simulink model "ES105A_StHlthSigNormn"  (R2013b)
settings: Solver=FixedStepDiscrete  SolverMode=SingleTasking  StartTime=0.0  StopTime=1  FixedStep=0.002  RelTol=1e-3
undefined symbols (not defined in the file): ARCHGLBPRM_FLOATZEROTHD_ULS_F32, CurrMeasCorrlnMaxErrCurr, CURRMOTSUMDIVBYZEROPROTNVAL_AMPR_F32, DIGTQDIVBYZEROPROTNVAL_HWNWTMTR_F32, DutyCycThermProtnDutyCycFildThd, EcuTMeasRngDiagcMax, EcuTMeasRngDiagcMin, EotLrngAuthyStrtLrn, FRICESTIMNDIVBYZEROPROTNVAL_HWNWTMTR_F32, HLTH0PERC_CNT_U08, HLTH100PERC_CNT_F32, HLTH100PERC_CNT_U08, HLTH50PERC_CNT_U08, HwTqCorrlnChATraSumSetFltThd, HwTqCorrlnChBTraSumSetFltThd, HWTQIDPTSIG_CNT_U08, MOTAG2MEAS_VALMAXERR_VOLTSQD_F32, MOTAG2MEAS_VALMINERR_VOLTSQD_F32, MOTAGCORRLN_MOTAGCORRLNERRTHD_MOTREVELEC_U0P16, MotDrvDiagcErrThd, MOTPOS2DIVBYZEROPROTNVAL2_VOLTSQD_F32, MOTPOS2DIVBYZEROPROTNVAL_VOLTSQD_F32, MOTPOSNERRDIVBYZEROPROTNVAL_MOTREV_U16, MOTPOSNERRZEROTHD_MOTREV_U0P16, NtcNr1, NtcSts1, PHAVLTGDIVBYZEROPROTNVAL_NANOSEC_F32, SigQlfr1, STHLTHSCAGFAC_CNT_F32, StHlthSigNormnAbsltMotPosDifStHlthDiagThd, StHlthSigNormnCurrMotSumStHlthDiagThd, StHlthSigNormnDigTqStHlthDiagThd, StHlthSigNormnDutyCycFltLimThd, StHlthSigNormnHiCtrlrT, StHlthSigNormnIdptSigStHlthSca, StHlthSigNormnLoCtrlrT, StHlthSigNormnMaxFricThd, StHlthSigNormnMinRackTrvlLim, StHlthSigNormnMotPosStHlthDiagThd, StHlthSigNormnMotVelCal, StHlthSigNormnPhaInfoStHlthDiagThd, StHlthSigNormnStHlthCorrlnErr, StHlthSigNormnStHlthCurrMotSum, StHlthSigNormnStHlthPhaInfo, StHlthSigNormnValMaxStHlthErr, StHlthSigNormnValMinStHlthErr, StHlthSigNormnWhlImbRejctnThd, SysGlbPrmMotPoleCnt, TSTHLTH0PERC_CNT_U08, u2, u3, u4, VLTGSTHLTH0PERC_CNT_U08
libraries: NxtrLim x39, simulink x33, NxtrAbslt x4
(part 5 of 10)

== system ES105A_StHlthSigNormn/StHlthSigNormn/UpdRawSig/Motor Position Error /AbsltMotPosBCDifStHlth Calc ==
  MotAgBCErrTerm : Inport
  Action Port : ActionPort  ActionType=default
  Constant4 : Constant  Value=StHlthSigNormnStHlthCorrlnErr
  CopyRight2 : Subsystem  Description=|  mask(Copyright Information){none=on}
      | Copyright info block.                                               
      |                                                                     
      | Place copyright information at the top of every subsystem in design.
      mask prompts: none "No parameters"
      mask help: Place copyright information at the top of every subsystem in design.
      mask Display:
      | NxtrConf = 'Nexteer Confidential';
      | 
      | sys = bdroot; %handle for the current model ("system")
      | first = get_param(sys,'Created');
      | first = first(end-3:end);  %year is last four digits
      | 
      | last = get_param(sys,'LastModifiedDate');
      | if isempty(last)
      |     last = datestr(now,'yyyy');
      | else
      |     last = last(end-3:end);
      | end
      | 
      | if strcmp(first,last)
      |     fprintf('%s -- Copyright %s Nexteer',NxtrConf,first)
      | else
      |     fprintf('%s -- %s%s- %s Nexteer',NxtrConf,char(169),first,last)
      | end
  If Action Subsystem8 : Subsystem  TreatAsAtomicUnit=on
  If Action Subsystem9 : Subsystem  TreatAsAtomicUnit=on
  If4 : If  IfExpression=u1
  LimStat_u3 : NxtrLim/LimStat_u08  LoLim=AbsltMotPosBCDifStHlth.EngMin  HiLim=AbsltMotPosBCDifStHlth.EngMax
      settings: AttributesFormatString=|
      | Low Limit: %<LoLim>
      | High Limit:%<HiLim>
  Merge2 : Merge
  Relational Operator4 : RelationalOperator  Operator=>  OutDataTypeStr=boolean
  AbsltMotPosBCDifStHlth : Outport  InitialOutput=HLTH100PERC_CNT_U08
      settings: AttributesFormatString=Initial Output: %<InitialOutput>
  wires:
  MotAgBCErrTerm/1 -> [MotAgBCErrTerm], Relational Operator4/1
  Constant4/1 -> Relational Operator4/2
  Relational Operator4/1 -> If4/1
  If4/1 -> If Action Subsystem8/Action
  If4/2 -> If Action Subsystem9/Action
  [MotAgBCErrTerm] -> If Action Subsystem8/1(MotAgBCErrTerm)
  If Action Subsystem8/1(AbsltMotPosBCDiffStHlth) -> Merge2/1
  If Action Subsystem9/1(AbsMotPosBCDiffStHlth) -> Merge2/2
  Merge2/1 -> LimStat_u3/1
  LimStat_u3/1 -> AbsltMotPosBCDifStHlth/1

== system ES105A_StHlthSigNormn/StHlthSigNormn/UpdRawSig/Motor Position Error /AbsltMotPosPhaDifStHlth ==
  NtcNr : Inport
  NtcStInfo : Inport  Port=2
  NtcSts : Inport  Port=3
  DebStep : Inport  Port=4
  SetNtcSts : Subsystem  RequirementInfo={} %GIDa_9ce26d92_e01b_4533_9a71_48efc3340490  TreatAsAtomicUnit=on
      settings: RTWSystemCode=Inline
  wires:
  NtcNr/1 -> SetNtcSts/1(NtcNr)  "NtcNr"
  NtcSts/1 -> SetNtcSts/3(NtcSts)
  DebStep/1 -> SetNtcSts/4(DebStep)
  NtcStInfo/1 -> SetNtcSts/2(NtcStInfo)

== system ES105A_StHlthSigNormn/StHlthSigNormn/UpdRawSig/Motor Position Error /CopyRight2 ==

== system ES105A_StHlthSigNormn/StHlthSigNormn/UpdRawSig/Motor Position Error /NTC Sts Calculation ==
  StHlthErr : Inport
  CopyRight2 : Subsystem  Description=|  mask(Copyright Information){none=on}
      | Copyright info block.                                               
      |                                                                     
      | Place copyright information at the top of every subsystem in design.
      mask prompts: none "No parameters"
      mask help: Place copyright information at the top of every subsystem in design.
      mask Display:
      | NxtrConf = 'Nexteer Confidential';
      | 
      | sys = bdroot; %handle for the current model ("system")
      | first = get_param(sys,'Created');
      | first = first(end-3:end);  %year is last four digits
      | 
      | last = get_param(sys,'LastModifiedDate');
      | if isempty(last)
      |     last = datestr(now,'yyyy');
      | else
      |     last = last(end-3:end);
      | end
      | 
      | if strcmp(first,last)
      |     fprintf('%s -- Copyright %s Nexteer',NxtrConf,first)
      | else
      |     fprintf('%s -- %s%s- %s Nexteer',NxtrConf,char(169),first,last)
      | end
  If : If  IfExpression=u1
  Merge : Merge
  NtcFaild : Subsystem  TreatAsAtomicUnit=on
  NtcPassd : Subsystem  TreatAsAtomicUnit=on
  NtcSts : Outport
  wires:
  StHlthErr/1 -> If/1
  If/1 -> NtcFaild/Action
  Merge/1 -> NtcSts/1
  NtcPassd/1(NtcPassd) -> Merge/2
  If/2 -> NtcPassd/Action
  NtcFaild/1(NtcFaild) -> Merge/1

== system ES105A_StHlthSigNormn/StHlthSigNormn/UpdRawSig/Phase Voltage Verification/CopyRight2 ==

== system ES105A_StHlthSigNormn/StHlthSigNormn/UpdRawSig/Phase Voltage Verification/NTC Sts Calculation ==
  StHlthErr : Inport
  CopyRight2 : Subsystem  Description=|  mask(Copyright Information){none=on}
      | Copyright info block.                                               
      |                                                                     
      | Place copyright information at the top of every subsystem in design.
      mask prompts: none "No parameters"
      mask help: Place copyright information at the top of every subsystem in design.
      mask Display:
      | NxtrConf = 'Nexteer Confidential';
      | 
      | sys = bdroot; %handle for the current model ("system")
      | first = get_param(sys,'Created');
      | first = first(end-3:end);  %year is last four digits
      | 
      | last = get_param(sys,'LastModifiedDate');
      | if isempty(last)
      |     last = datestr(now,'yyyy');
      | else
      |     last = last(end-3:end);
      | end
      | 
      | if strcmp(first,last)
      |     fprintf('%s -- Copyright %s Nexteer',NxtrConf,first)
      | else
      |     fprintf('%s -- %s%s- %s Nexteer',NxtrConf,char(169),first,last)
      | end
  If : If  IfExpression=u1
  Merge : Merge
  NtcFaild : Subsystem  TreatAsAtomicUnit=on
  NtcPassd : Subsystem  TreatAsAtomicUnit=on
  NtcSts : Outport
  wires:
  StHlthErr/1 -> If/1
  If/1 -> NtcFaild/Action
  Merge/1 -> NtcSts/1
  NtcPassd/1(NtcPassd) -> Merge/2
  If/2 -> NtcPassd/Action
  NtcFaild/1(NtcFaild) -> Merge/1

== system ES105A_StHlthSigNormn/StHlthSigNormn/UpdRawSig/Phase Voltage Verification/PhaAStHlth Calc ==
  MotDrvErrA : Inport
  Action Port : ActionPort  ActionType=case
  Constant : Constant  Value=StHlthSigNormnStHlthPhaInfo
  CopyRight2 : Subsystem  Description=|  mask(Copyright Information){none=on}
      | Copyright info block.                                               
      |                                                                     
      | Place copyright information at the top of every subsystem in design.
      mask prompts: none "No parameters"
      mask help: Place copyright information at the top of every subsystem in design.
      mask Display:
      | NxtrConf = 'Nexteer Confidential';
      | 
      | sys = bdroot; %handle for the current model ("system")
      | first = get_param(sys,'Created');
      | first = first(end-3:end);  %year is last four digits
      | 
      | last = get_param(sys,'LastModifiedDate');
      | if isempty(last)
      |     last = datestr(now,'yyyy');
      | else
      |     last = last(end-3:end);
      | end
      | 
      | if strcmp(first,last)
      |     fprintf('%s -- Copyright %s Nexteer',NxtrConf,first)
      | else
      |     fprintf('%s -- %s%s- %s Nexteer',NxtrConf,char(169),first,last)
      | end
  If : If  IfExpression=u1
  If Action Subsystem : Subsystem  TreatAsAtomicUnit=on
  If Action Subsystem1 : Subsystem  TreatAsAtomicUnit=on
  LimStat_u2 : NxtrLim/LimStat_u08  LoLim=PhaAStHlth.EngMin  HiLim=PhaAStHlth.EngMax
      settings: AttributesFormatString=|
      | Low Limit: %<LoLim>
      | High Limit:%<HiLim>
  Merge : Merge
  Relational Operator : RelationalOperator  Operator=>  OutDataTypeStr=boolean
  PhaAStHlth : Outport  InitialOutput=HLTH100PERC_CNT_U08
      settings: AttributesFormatString=Initial Output: %<InitialOutput>
  wires:
  MotDrvErrA/1 -> [MotDrvErrA], Relational Operator/1
  Constant/1 -> Relational Operator/2
  Relational Operator/1 -> If/1
  If/1 -> If Action Subsystem/Action
  If/2 -> If Action Subsystem1/Action
  [MotDrvErrA] -> If Action Subsystem/1(MotDrvErrA)
  If Action Subsystem/1(PhaseAStHlth) -> Merge/1
  If Action Subsystem1/1(PhaseAStHlth) -> Merge/2
  LimStat_u2/1 -> PhaAStHlth/1
  Merge/1 -> LimStat_u2/1

== system ES105A_StHlthSigNormn/StHlthSigNormn/UpdRawSig/Phase Voltage Verification/PhaBStHlth Calc ==
  MotDrvErrB : Inport
  Action Port : ActionPort  ActionType=case
  Constant2 : Constant  Value=StHlthSigNormnStHlthPhaInfo
  CopyRight2 : Subsystem  Description=|  mask(Copyright Information){none=on}
      | Copyright info block.                                               
      |                                                                     
      | Place copyright information at the top of every subsystem in design.
      mask prompts: none "No parameters"
      mask help: Place copyright information at the top of every subsystem in design.
      mask Display:
      | NxtrConf = 'Nexteer Confidential';
      | 
      | sys = bdroot; %handle for the current model ("system")
      | first = get_param(sys,'Created');
      | first = first(end-3:end);  %year is last four digits
      | 
      | last = get_param(sys,'LastModifiedDate');
      | if isempty(last)
      |     last = datestr(now,'yyyy');
      | else
      |     last = last(end-3:end);
      | end
      | 
      | if strcmp(first,last)
      |     fprintf('%s -- Copyright %s Nexteer',NxtrConf,first)
      | else
      |     fprintf('%s -- %s%s- %s Nexteer',NxtrConf,char(169),first,last)
      | end
  If Action Subsystem4 : Subsystem  TreatAsAtomicUnit=on
  If Action Subsystem5 : Subsystem  TreatAsAtomicUnit=on
  If2 : If  IfExpression=u1
  LimStat_u1 : NxtrLim/LimStat_u08  LoLim=PhaBStHlth.EngMin  HiLim=PhaBStHlth.EngMax
      settings: AttributesFormatString=|
      | Low Limit: %<LoLim>
      | High Limit:%<HiLim>
  Merge1 : Merge
  Relational Operator2 : RelationalOperator  Operator=>  OutDataTypeStr=boolean
  PhaBStHlth : Outport  InitialOutput=HLTH100PERC_CNT_U08
      settings: AttributesFormatString=Initial Output: %<InitialOutput>
  wires:
  MotDrvErrB/1 -> [MotDrvErrB], Relational Operator2/1
  Constant2/1 -> Relational Operator2/2
  Relational Operator2/1 -> If2/1
  If2/1 -> If Action Subsystem4/Action
  If2/2 -> If Action Subsystem5/Action
  [MotDrvErrB] -> If Action Subsystem4/1(MotDrvErrB)
  If Action Subsystem4/1(PhaseBStHlth) -> Merge1/1
  If Action Subsystem5/1(PhaseAStHlth) -> Merge1/2
  Merge1/1 -> LimStat_u1/1
  LimStat_u1/1 -> PhaBStHlth/1

== system ES105A_StHlthSigNormn/StHlthSigNormn/UpdRawSig/Phase Voltage Verification/PhaCStHlth Calc ==
  MotDrvErrC : Inport
  Action Port : ActionPort  ActionType=case
  Constant4 : Constant  Value=StHlthSigNormnStHlthPhaInfo
  CopyRight2 : Subsystem  Description=|  mask(Copyright Information){none=on}
      | Copyright info block.                                               
      |                                                                     
      | Place copyright information at the top of every subsystem in design.
      mask prompts: none "No parameters"
      mask help: Place copyright information at the top of every subsystem in design.
      mask Display:
      | NxtrConf = 'Nexteer Confidential';
      | 
      | sys = bdroot; %handle for the current model ("system")
      | first = get_param(sys,'Created');
      | first = first(end-3:end);  %year is last four digits
      | 
      | last = get_param(sys,'LastModifiedDate');
      | if isempty(last)
      |     last = datestr(now,'yyyy');
      | else
      |     last = last(end-3:end);
      | end
      | 
      | if strcmp(first,last)
      |     fprintf('%s -- Copyright %s Nexteer',NxtrConf,first)
      | else
      |     fprintf('%s -- %s%s- %s Nexteer',NxtrConf,char(169),first,last)
      | end
  If Action Subsystem8 : Subsystem  TreatAsAtomicUnit=on
  If Action Subsystem9 : Subsystem  TreatAsAtomicUnit=on
  If4 : If  IfExpression=u1
  LimStat_u3 : NxtrLim/LimStat_u08  LoLim=PhaCStHlth.EngMin  HiLim=PhaCStHlth.EngMax
      settings: AttributesFormatString=|
      | Low Limit: %<LoLim>
      | High Limit:%<HiLim>
  Merge2 : Merge
  Relational Operator4 : RelationalOperator  Operator=>  OutDataTypeStr=boolean
  PhaCStHlth : Outport  InitialOutput=HLTH100PERC_CNT_U08
      settings: AttributesFormatString=Initial Output: %<InitialOutput>
  wires:
  MotDrvErrC/1 -> [MotDrvErrC], Relational Operator4/1
  Constant4/1 -> Relational Operator4/2
  Relational Operator4/1 -> If4/1
  If4/1 -> If Action Subsystem8/Action
  If4/2 -> If Action Subsystem9/Action
  [MotDrvErrC] -> If Action Subsystem8/1(MotDrvErrC)
  If Action Subsystem8/1(PhaseCStHlth) -> Merge2/1
  If Action Subsystem9/1(PhaseCStHlth) -> Merge2/2
  Merge2/1 -> LimStat_u3/1
  LimStat_u3/1 -> PhaCStHlth/1

== system ES105A_StHlthSigNormn/StHlthSigNormn/UpdRawSig/Phase Voltage Verification/PhaDStHlth Calc ==
  MotDrvErrD : Inport
  Action Port : ActionPort  ActionType=case
  Constant6 : Constant  Value=StHlthSigNormnStHlthPhaInfo
  CopyRight2 : Subsystem  Description=|  mask(Copyright Information){none=on}
      | Copyright info block.                                               
      |                                                                     
      | Place copyright information at the top of every subsystem in design.
      mask prompts: none "No parameters"
      mask help: Place copyright information at the top of every subsystem in design.
      mask Display:
      | NxtrConf = 'Nexteer Confidential';
      | 
      | sys = bdroot; %handle for the current model ("system")
      | first = get_param(sys,'Created');
      | first = first(end-3:end);  %year is last four digits
      | 
      | last = get_param(sys,'LastModifiedDate');
      | if isempty(last)
      |     last = datestr(now,'yyyy');
      | else
      |     last = last(end-3:end);
      | end
      | 
      | if strcmp(first,last)
      |     fprintf('%s -- Copyright %s Nexteer',NxtrConf,first)
      | else
      |     fprintf('%s -- %s%s- %s Nexteer',NxtrConf,char(169),first,last)
      | end
  If Action Subsystem12 : Subsystem  TreatAsAtomicUnit=on
  If Action Subsystem13 : Subsystem  TreatAsAtomicUnit=on
  If6 : If  IfExpression=u1
  LimStat_u4 : NxtrLim/LimStat_u08  LoLim=PhaDStHlth.EngMin  HiLim=PhaDStHlth.EngMax
      settings: AttributesFormatString=|
      | Low Limit: %<LoLim>
      | High Limit:%<HiLim>
  Merge3 : Merge
  Relational Operator6 : RelationalOperator  Operator=>  OutDataTypeStr=boolean
  PhaDStHlth : Outport  InitialOutput=HLTH100PERC_CNT_U08
      settings: AttributesFormatString=Initial Output: %<InitialOutput>
  wires:
  MotDrvErrD/1 -> [MotDrvErrD], Relational Operator6/1
  Constant6/1 -> Relational Operator6/2
  Relational Operator6/1 -> If6/1
  If6/1 -> If Action Subsystem12/Action
  If6/2 -> If Action Subsystem13/Action
  [MotDrvErrD] -> If Action Subsystem12/1(MotDrvErrD)
  If Action Subsystem12/1(PhaseDStHlth) -> Merge3/1
  If Action Subsystem13/1(PhaseDStHlth) -> Merge3/2
  Merge3/1 -> LimStat_u4/1
  LimStat_u4/1 -> PhaDStHlth/1

== system ES105A_StHlthSigNormn/StHlthSigNormn/UpdRawSig/Phase Voltage Verification/PhaEStHlth Calc ==
  MotDrvErrE : Inport
  Action Port : ActionPort  ActionType=case
  Constant8 : Constant  Value=StHlthSigNormnStHlthPhaInfo
  CopyRight2 : Subsystem  Description=|  mask(Copyright Information){none=on}
      | Copyright info block.                                               
      |                                                                     
      | Place copyright information at the top of every subsystem in design.
      mask prompts: none "No parameters"
      mask help: Place copyright information at the top of every subsystem in design.
      mask Display:
      | NxtrConf = 'Nexteer Confidential';
      | 
      | sys = bdroot; %handle for the current model ("system")
      | first = get_param(sys,'Created');
      | first = first(end-3:end);  %year is last four digits
      | 
      | last = get_param(sys,'LastModifiedDate');
      | if isempty(last)
      |     last = datestr(now,'yyyy');
      | else
      |     last = last(end-3:end);
      | end
      | 
      | if strcmp(first,last)
      |     fprintf('%s -- Copyright %s Nexteer',NxtrConf,first)
      | else
      |     fprintf('%s -- %s%s- %s Nexteer',NxtrConf,char(169),first,last)
      | end
  If Action Subsystem16 : Subsystem  TreatAsAtomicUnit=on
  If Action Subsystem17 : Subsystem  TreatAsAtomicUnit=on
  If8 : If  IfExpression=u1
  LimStat_u5 : NxtrLim/LimStat_u08  LoLim=PhaEStHlth.EngMin  HiLim=PhaEStHlth.EngMax
      settings: AttributesFormatString=|
      | Low Limit: %<LoLim>
      | High Limit:%<HiLim>
  Merge4 : Merge
  Relational Operator8 : RelationalOperator  Operator=>  OutDataTypeStr=boolean
  PhaEStHlth : Outport  InitialOutput=HLTH100PERC_CNT_U08
      settings: AttributesFormatString=Initial Output: %<InitialOutput>
  wires:
  MotDrvErrE/1 -> [MotDrvErrE], Relational Operator8/1
  Constant8/1 -> Relational Operator8/2
  Relational Operator8/1 -> If8/1
  If8/1 -> If Action Subsystem16/Action
  If8/2 -> If Action Subsystem17/Action
  [MotDrvErrE] -> If Action Subsystem16/1(MotDrvErrE)
  If Action Subsystem16/1(PhaseEStHlth) -> Merge4/1
  If Action Subsystem17/1(PhaseEStHlth) -> Merge4/2
  Merge4/1 -> LimStat_u5/1
  LimStat_u5/1 -> PhaEStHlth/1

== system ES105A_StHlthSigNormn/StHlthSigNormn/UpdRawSig/Phase Voltage Verification/PhaFStHlth Calc ==
  MotDrvErrF : Inport
  Action Port : ActionPort  ActionType=default
  Constant10 : Constant  Value=StHlthSigNormnStHlthPhaInfo
  CopyRight2 : Subsystem  Description=|  mask(Copyright Information){none=on}
      | Copyright info block.                                               
      |                                                                     
      | Place copyright information at the top of every subsystem in design.
      mask prompts: none "No parameters"
      mask help: Place copyright information at the top of every subsystem in design.
      mask Display:
      | NxtrConf = 'Nexteer Confidential';
      | 
      | sys = bdroot; %handle for the current model ("system")
      | first = get_param(sys,'Created');
      | first = first(end-3:end);  %year is last four digits
      | 
      | last = get_param(sys,'LastModifiedDate');
      | if isempty(last)
      |     last = datestr(now,'yyyy');
      | else
      |     last = last(end-3:end);
      | end
      | 
      | if strcmp(first,last)
      |     fprintf('%s -- Copyright %s Nexteer',NxtrConf,first)
      | else
      |     fprintf('%s -- %s%s- %s Nexteer',NxtrConf,char(169),first,last)
      | end
  If Action Subsystem20 : Subsystem  TreatAsAtomicUnit=on
  If Action Subsystem21 : Subsystem  TreatAsAtomicUnit=on
  If10 : If  IfExpression=u1
  LimStat_u6 : NxtrLim/LimStat_u08  LoLim=PhaFStHlth.EngMin  HiLim=PhaFStHlth.EngMax
      settings: AttributesFormatString=|
      | Low Limit: %<LoLim>
      | High Limit:%<HiLim>
  Merge5 : Merge
  Relational Operator10 : RelationalOperator  Operator=>  OutDataTypeStr=boolean
  PhaFStHlth : Outport  InitialOutput=HLTH100PERC_CNT_U08
      settings: AttributesFormatString=Initial Output: %<InitialOutput>
  wires:
  MotDrvErrF/1 -> [MotDrvErrF], Relational Operator10/1
  Constant10/1 -> Relational Operator10/2
  Relational Operator10/1 -> If10/1
  If10/1 -> If Action Subsystem20/Action
  If10/2 -> If Action Subsystem21/Action
  [MotDrvErrF] -> If Action Subsystem20/1(MotDrvErrF)
  If Action Subsystem20/1(PhaseFStHlth) -> Merge5/1
  If Action Subsystem21/1(PhaseFStHlth) -> Merge5/2
  LimStat_u6/1 -> PhaFStHlth/1
  Merge5/1 -> LimStat_u6/1

== system ES105A_StHlthSigNormn/StHlthSigNormn/UpdRawSig/Phase Voltage Verification/PhaStHlth ==
  NtcNr : Inport
  NtcStInfo : Inport  Port=2
  NtcSts : Inport  Port=3
  DebStep : Inport  Port=4
  SetNtcSts : Subsystem  RequirementInfo={} %GIDa_c9812cd9_0524_4ca1_aa4b_483209325d77  TreatAsAtomicUnit=on
      settings: RTWSystemCode=Inline
  wires:
  NtcNr/1 -> SetNtcSts/1(NtcNr)  "NtcNr"
  NtcSts/1 -> SetNtcSts/3(NtcSts)
  DebStep/1 -> SetNtcSts/4(DebStep)
  NtcStInfo/1 -> SetNtcSts/2(NtcStInfo)

== system ES105A_StHlthSigNormn/StHlthSigNormn/UpdRawSig/Single Bit Correction /CopyRight2 ==

== system ES105A_StHlthSigNormn/StHlthSigNormn/UpdRawSig/Wheel Imbalance Rejection/CopyRight2 ==

== system ES105A_StHlthSigNormn/StHlthSigNormn/UpdRawSig/Wheel Imbalance Rejection/If Action Subsystem ==
  Action Port : ActionPort  ActionType=then
  Constant : Constant  Value=HLTH0PERC_CNT_U08
  CopyRight2 : Subsystem  Description=|  mask(Copyright Information){none=on}
      | Copyright info block.                                               
      |                                                                     
      | Place copyright information at the top of every subsystem in design.
      mask prompts: none "No parameters"
      mask help: Place copyright information at the top of every subsystem in design.
      mask Display:
      | NxtrConf = 'Nexteer Confidential';
      | 
      | sys = bdroot; %handle for the current model ("system")
      | first = get_param(sys,'Created');
      | first = first(end-3:end);  %year is last four digits
      | 
      | last = get_param(sys,'LastModifiedDate');
      | if isempty(last)
      |     last = datestr(now,'yyyy');
      | else
      |     last = last(end-3:end);
      | end
      | 
      | if strcmp(first,last)
      |     fprintf('%s -- Copyright %s Nexteer',NxtrConf,first)
      | else
      |     fprintf('%s -- %s%s- %s Nexteer',NxtrConf,char(169),first,last)
      | end
  WhlImbMaxCmpStHlth : Outport
  wires:
  Constant/1 -> WhlImbMaxCmpStHlth/1

== system ES105A_StHlthSigNormn/StHlthSigNormn/UpdRawSig/Wheel Imbalance Rejection/If Action Subsystem2 ==
  Action Port : ActionPort  ActionType=else
  Constant : Constant  Value=HLTH100PERC_CNT_U08
  CopyRight2 : Subsystem  Description=|  mask(Copyright Information){none=on}
      | Copyright info block.                                               
      |                                                                     
      | Place copyright information at the top of every subsystem in design.
      mask prompts: none "No parameters"
      mask help: Place copyright information at the top of every subsystem in design.
      mask Display:
      | NxtrConf = 'Nexteer Confidential';
      | 
      | sys = bdroot; %handle for the current model ("system")
      | first = get_param(sys,'Created');
      | first = first(end-3:end);  %year is last four digits
      | 
      | last = get_param(sys,'LastModifiedDate');
      | if isempty(last)
      |     last = datestr(now,'yyyy');
      | else
      |     last = last(end-3:end);
      | end
      | 
      | if strcmp(first,last)
      |     fprintf('%s -- Copyright %s Nexteer',NxtrConf,first)
      | else
      |     fprintf('%s -- %s%s- %s Nexteer',NxtrConf,char(169),first,last)
      | end
  WhlImbMaxCmpStHlth : Outport
  wires:
  Constant/1 -> WhlImbMaxCmpStHlth/1

== system ES105A_StHlthSigNormn/StHlthSigNormn/UpdRawSig/ EOT Impact Counter/If Action Subsystem/CopyRight2 ==

== system ES105A_StHlthSigNormn/StHlthSigNormn/UpdRawSig/ EOT Impact Counter/If Action Subsystem/If Action Subsystem ==
  RackLimrEotSig1Avl : Inport
  HwAg : Inport  Port=2
  "MotVelCrf " : Inport  Port=3
  HwAgEotCw : Inport  Port=4
  Action Port : ActionPort  ActionType=then
  Add : Sum  Inputs=+-
  Constant1 : Constant  Value=StHlthSigNormnMinRackTrvlLim
  CopyRight2 : Subsystem  Description=|  mask(Copyright Information){none=on}
      | Copyright info block.                                               
      |                                                                     
      | Place copyright information at the top of every subsystem in design.
      mask prompts: none "No parameters"
      mask help: Place copyright information at the top of every subsystem in design.
      mask Display:
      | NxtrConf = 'Nexteer Confidential';
      | 
      | sys = bdroot; %handle for the current model ("system")
      | first = get_param(sys,'Created');
      | first = first(end-3:end);  %year is last four digits
      | 
      | last = get_param(sys,'LastModifiedDate');
      | if isempty(last)
      |     last = datestr(now,'yyyy');
      | else
      |     last = last(end-3:end);
      | end
      | 
      | if strcmp(first,last)
      |     fprintf('%s -- Copyright %s Nexteer',NxtrConf,first)
      | else
      |     fprintf('%s -- %s%s- %s Nexteer',NxtrConf,char(169),first,last)
      | end
  If : If  IfExpression=u1
  If Action Subsystem : Subsystem  TreatAsAtomicUnit=on
  If Action Subsystem1 : Subsystem  TreatAsAtomicUnit=on
  Logical Operator : Logic  AllPortsSameDT=off  OutDataTypeStr=boolean
  Relational Operator1 : RelationalOperator  OutDataTypeStr=boolean
  wires:
  HwAg/1 -> Relational Operator1/1
  RackLimrEotSig1Avl/1 -> Logical Operator/1
  Relational Operator1/1 -> Logical Operator/2
  Add/1 -> Relational Operator1/2
  Logical Operator/1 -> If/1
  If/1 -> If Action Subsystem/Action
  If/2 -> If Action Subsystem1/Action
  "MotVelCrf "/1 -> If Action Subsystem/1("MotVelCrf ")
  HwAgEotCw/1 -> Add/1
  Constant1/1 -> Add/2

== system ES105A_StHlthSigNormn/StHlthSigNormn/UpdRawSig/ EOT Impact Counter/If Action Subsystem/If Action Subsystem1 ==
  RackLimrEotSig0Avl : Inport
  HwAg : Inport  Port=2
  MotVelCrf : Inport  Port=3
  HwAgEotCcw : Inport  Port=4
  Action Port : ActionPort  ActionType=else
  Add : Sum
  Constant1 : Constant  Value=StHlthSigNormnMinRackTrvlLim
  CopyRight2 : Subsystem  Description=|  mask(Copyright Information){none=on}
      | Copyright info block.                                               
      |                                                                     
      | Place copyright information at the top of every subsystem in design.
      mask prompts: none "No parameters"
      mask help: Place copyright information at the top of every subsystem in design.
      mask Display:
      | NxtrConf = 'Nexteer Confidential';
      | 
      | sys = bdroot; %handle for the current model ("system")
      | first = get_param(sys,'Created');
      | first = first(end-3:end);  %year is last four digits
      | 
      | last = get_param(sys,'LastModifiedDate');
      | if isempty(last)
      |     last = datestr(now,'yyyy');
      | else
      |     last = last(end-3:end);
      | end
      | 
      | if strcmp(first,last)
      |     fprintf('%s -- Copyright %s Nexteer',NxtrConf,first)
      | else
      |     fprintf('%s -- %s%s- %s Nexteer',NxtrConf,char(169),first,last)
      | end
  If : If  IfExpression=u1
  If Action Subsystem : Subsystem  TreatAsAtomicUnit=on
  If Action Subsystem1 : Subsystem  TreatAsAtomicUnit=on
  Logical Operator : Logic  AllPortsSameDT=off  OutDataTypeStr=boolean
  Relational Operator1 : RelationalOperator  Operator=<=  OutDataTypeStr=boolean
  wires:
  HwAg/1 -> Relational Operator1/1
  RackLimrEotSig0Avl/1 -> Logical Operator/1
  Relational Operator1/1 -> Logical Operator/2
  Add/1 -> Relational Operator1/2
  Logical Operator/1 -> If/1
  If/1 -> If Action Subsystem/Action
  If/2 -> If Action Subsystem1/Action
  MotVelCrf/1 -> If Action Subsystem/1("MotVelCrf ")
  Constant1/1 -> Add/2
  HwAgEotCcw/1 -> Add/1

== system ES105A_StHlthSigNormn/StHlthSigNormn/UpdRawSig/ EOT Impact Counter/If Action Subsystem1/CopyRight2 ==

== system ES105A_StHlthSigNormn/StHlthSigNormn/UpdRawSig/ Health Of Assist Due To Voltage/Do nothing/CopyRight2 ==

== system ES105A_StHlthSigNormn/StHlthSigNormn/UpdRawSig/ Health Of Assist Due To Voltage/LowVoltage/CopyRight2 ==

== system ES105A_StHlthSigNormn/StHlthSigNormn/UpdRawSig/ Health Of Assist Due To Voltage/NtcLoVltgActvSts/CopyRight2 ==

== system ES105A_StHlthSigNormn/StHlthSigNormn/UpdRawSig/ Health Of Assist Due To Voltage/NtcOverVltgActvSts/CopyRight2 ==

== system ES105A_StHlthSigNormn/StHlthSigNormn/UpdRawSig/ Health Of Assist Due To Voltage/NtcUnderVltgActvSts/CopyRight2 ==

== system ES105A_StHlthSigNormn/StHlthSigNormn/UpdRawSig/ Health Of Assist Due To Voltage/OverVoltage/CopyRight2 ==

== system ES105A_StHlthSigNormn/StHlthSigNormn/UpdRawSig/ Health Of Assist Due To Voltage/Safe Operating Conditions/CopyRight2 ==

== system ES105A_StHlthSigNormn/StHlthSigNormn/UpdRawSig/ Health Of Assist Due To Voltage/UnderVoltage/CopyRight2 ==

== system ES105A_StHlthSigNormn/StHlthSigNormn/UpdRawSig/ Health Of Assist Due To Voltage/Voltage range update for ignition cycle/CopyRight2 ==

== system ES105A_StHlthSigNormn/StHlthSigNormn/UpdRawSig/ Health Of Assist Due To Voltage/Voltage range update for ignition cycle1/CopyRight2 ==

== system ES105A_StHlthSigNormn/StHlthSigNormn/UpdRawSig/ Health Of Assist Due To Voltage/Voltage range update for present cycle /CopyRight2 ==

== system ES105A_StHlthSigNormn/StHlthSigNormn/UpdRawSig/ Health Of Assist Due To Voltage/Voltage range update for present cycle1/CopyRight2 ==

== system ES105A_StHlthSigNormn/StHlthSigNormn/UpdRawSig/Controller temperature/Controller temperature range update for ignition cycle/CopyRight2 ==

== system ES105A_StHlthSigNormn/StHlthSigNormn/UpdRawSig/Controller temperature/Controller temperature range update for ignition cycle1/CopyRight2 ==

== system ES105A_StHlthSigNormn/StHlthSigNormn/UpdRawSig/Controller temperature/Controller temperature range update for present cycle /CopyRight2 ==

== system ES105A_StHlthSigNormn/StHlthSigNormn/UpdRawSig/Controller temperature/Controller temperature range update for present cycle1/CopyRight2 ==

== system ES105A_StHlthSigNormn/StHlthSigNormn/UpdRawSig/Controller temperature/CtrlrTStHlth0Perc/CopyRight2 ==

== system ES105A_StHlthSigNormn/StHlthSigNormn/UpdRawSig/Controller temperature/CtrlrTStHlth0Perc1/CopyRight2 ==

== system ES105A_StHlthSigNormn/StHlthSigNormn/UpdRawSig/Controller temperature/CtrlrTStHlth100Perc/CopyRight2 ==

== system ES105A_StHlthSigNormn/StHlthSigNormn/UpdRawSig/Controller temperature/CtrlrTStHlth50Perc/CopyRight2 ==

== system ES105A_StHlthSigNormn/StHlthSigNormn/UpdRawSig/Controller temperature/CtrlrTStHlth50Perc1/CopyRight2 ==

== system ES105A_StHlthSigNormn/StHlthSigNormn/UpdRawSig/Current Error/CurrMotSumABCStHlth Calc/CopyRight2 ==

== system ES105A_StHlthSigNormn/StHlthSigNormn/UpdRawSig/Current Error/CurrMotSumABCStHlth Calc/If Action Subsystem ==
  CurrMotSumABC : Inport
  Action Port : ActionPort  ActionType=then
  Constant : Constant  Value=CurrMeasCorrlnMaxErrCurr
  CopyRight2 : Subsystem  Description=|  mask(Copyright Information){none=on}
      | Copyright info block.                                               
      |                                                                     
      | Place copyright information at the top of every subsystem in design.
      mask prompts: none "No parameters"
      mask help: Place copyright information at the top of every subsystem in design.
      mask Display:
      | NxtrConf = 'Nexteer Confidential';
      | 
      | sys = bdroot; %handle for the current model ("system")
      | first = get_param(sys,'Created');
      | first = first(end-3:end);  %year is last four digits
      | 
      | last = get_param(sys,'LastModifiedDate');
      | if isempty(last)
      |     last = datestr(now,'yyyy');
      | else
      |     last = last(end-3:end);
      | end
      | 
      | if strcmp(first,last)
      |     fprintf('%s -- Copyright %s Nexteer',NxtrConf,first)
      | else
      |     fprintf('%s -- %s%s- %s Nexteer',NxtrConf,char(169),first,last)
      | end
  If : If  IfExpression=u1
  If Action Subsystem : Subsystem  TreatAsAtomicUnit=on
  If Action Subsystem1 : Subsystem  TreatAsAtomicUnit=on
  Merge : Merge
  Relational Operator : RelationalOperator  OutDataTypeStr=boolean
  CurrMotSumABCStHlth : Outport
  wires:
  CurrMotSumABC/1 -> [CurrMotSumABC], Relational Operator/1
  Constant/1 -> Relational Operator/2
  Relational Operator/1 -> If/1
  If/1 -> If Action Subsystem/Action
  If/2 -> If Action Subsystem1/Action
  [CurrMotSumABC] -> If Action Subsystem1/1(CurrMotSumABC)
  If Action Subsystem/1(CurrMotSumABCStHlth) -> Merge/1
  If Action Subsystem1/1(CurrMotSumABCStHlth) -> Merge/2
  Merge/1 -> CurrMotSumABCStHlth/1

== system ES105A_StHlthSigNormn/StHlthSigNormn/UpdRawSig/Current Error/CurrMotSumABCStHlth Calc/If Action Subsystem1 ==
  Action Port : ActionPort  ActionType=else
  Constant : Constant  Value=HLTH100PERC_CNT_U08
  CopyRight2 : Subsystem  Description=|  mask(Copyright Information){none=on}
      | Copyright info block.                                               
      |                                                                     
      | Place copyright information at the top of every subsystem in design.
      mask prompts: none "No parameters"
      mask help: Place copyright information at the top of every subsystem in design.
      mask Display:
      | NxtrConf = 'Nexteer Confidential';
      | 
      | sys = bdroot; %handle for the current model ("system")
      | first = get_param(sys,'Created');
      | first = first(end-3:end);  %year is last four digits
      | 
      | last = get_param(sys,'LastModifiedDate');
      | if isempty(last)
      |     last = datestr(now,'yyyy');
      | else
      |     last = last(end-3:end);
      | end
      | 
      | if strcmp(first,last)
      |     fprintf('%s -- Copyright %s Nexteer',NxtrConf,first)
      | else
      |     fprintf('%s -- %s%s- %s Nexteer',NxtrConf,char(169),first,last)
      | end
  CurrMotSumABCStHlth : Outport
  wires:
  Constant/1 -> CurrMotSumABCStHlth/1

== system ES105A_StHlthSigNormn/StHlthSigNormn/UpdRawSig/Current Error/CurrMotSumDEFStHlth Calc/CopyRight2 ==

== system ES105A_StHlthSigNormn/StHlthSigNormn/UpdRawSig/Current Error/CurrMotSumDEFStHlth Calc/If Action Subsystem4 ==
  CurrMotSumDEF : Inport
  Action Port : ActionPort  ActionType=then
  Constant : Constant  Value=CurrMeasCorrlnMaxErrCurr
  CopyRight2 : Subsystem  Description=|  mask(Copyright Information){none=on}
      | Copyright info block.                                               
      |                                                                     
      | Place copyright information at the top of every subsystem in design.
      mask prompts: none "No parameters"
      mask help: Place copyright information at the top of every subsystem in design.
      mask Display:
      | NxtrConf = 'Nexteer Confidential';
      | 
      | sys = bdroot; %handle for the current model ("system")
      | first = get_param(sys,'Created');
      | first = first(end-3:end);  %year is last four digits
      | 
      | last = get_param(sys,'LastModifiedDate');
      | if isempty(last)
      |     last = datestr(now,'yyyy');
      | else
      |     last = last(end-3:end);
      | end
      | 
      | if strcmp(first,last)
      |     fprintf('%s -- Copyright %s Nexteer',NxtrConf,first)
      | else
      |     fprintf('%s -- %s%s- %s Nexteer',NxtrConf,char(169),first,last)
      | end
  If : If  IfExpression=u1
  If Action Subsystem : Subsystem  TreatAsAtomicUnit=on
  If Action Subsystem1 : Subsystem  TreatAsAtomicUnit=on
  Merge : Merge
  Relational Operator : RelationalOperator  OutDataTypeStr=boolean
  CurrMotSumDEFStHlth : Outport
  wires:
  CurrMotSumDEF/1 -> [CurrMotSumDEF], Relational Operator/1
  Constant/1 -> Relational Operator/2
  Relational Operator/1 -> If/1
  If/1 -> If Action Subsystem/Action
  If/2 -> If Action Subsystem1/Action
  [CurrMotSumDEF] -> If Action Subsystem1/1(CurrMotSumDEF)
  If Action Subsystem/1(CurrMotSumDEFStHlth) -> Merge/1
  If Action Subsystem1/1(CurrMotSumDEFStHlth) -> Merge/2
  Merge/1 -> CurrMotSumDEFStHlth/1

== system ES105A_StHlthSigNormn/StHlthSigNormn/UpdRawSig/Current Error/CurrMotSumDEFStHlth Calc/If Action Subsystem5 ==
  Action Port : ActionPort  ActionType=else
  Constant : Constant  Value=HLTH100PERC_CNT_U08
  CopyRight2 : Subsystem  Description=|  mask(Copyright Information){none=on}
      | Copyright info block.                                               
      |                                                                     
      | Place copyright information at the top of every subsystem in design.
      mask prompts: none "No parameters"
      mask help: Place copyright information at the top of every subsystem in design.
      mask Display:
      | NxtrConf = 'Nexteer Confidential';
      | 
      | sys = bdroot; %handle for the current model ("system")
      | first = get_param(sys,'Created');
      | first = first(end-3:end);  %year is last four digits
      | 
      | last = get_param(sys,'LastModifiedDate');
      | if isempty(last)
      |     last = datestr(now,'yyyy');
      | else
      |     last = last(end-3:end);
      | end
      | 
      | if strcmp(first,last)
      |     fprintf('%s -- Copyright %s Nexteer',NxtrConf,first)
      | else
      |     fprintf('%s -- %s%s- %s Nexteer',NxtrConf,char(169),first,last)
      | end
  CurrMotSumDEFStHlth : Outport
  wires:
  Constant/1 -> CurrMotSumDEFStHlth/1

== system ES105A_StHlthSigNormn/StHlthSigNormn/UpdRawSig/Current Error/CurrMotSumPhaStHlth/SetNtcSts ==
  note: Note:
      |
      | - "ISO Fault Debounce Design" Simulink block intent to use here for Simulation purpose only. Do not Code this block
  NtcNr : Inport
  NtcStInfo : Inport  Port=2
  NtcSts : Inport  Port=3
  DebStep : Inport  Port=4
  CopyRight2 : Subsystem  Description=|  mask(Copyright Information){none=on}
      | Copyright info block.                                               
      |                                                                     
      | Place copyright information at the top of every subsystem in design.
      mask prompts: none "No parameters"
      mask help: Place copyright information at the top of every subsystem in design.
      mask Display:
      | NxtrConf = 'Nexteer Confidential';
      | 
      | sys = bdroot; %handle for the current model ("system")
      | first = get_param(sys,'Created');
      | first = first(end-3:end);  %year is last four digits
      | 
      | last = get_param(sys,'LastModifiedDate');
      | if isempty(last)
      |     last = datestr(now,'yyyy');
      | else
      |     last = last(end-3:end);
      | end
      | 
      | if strcmp(first,last)
      |     fprintf('%s -- Copyright %s Nexteer',NxtrConf,first)
      | else
      |     fprintf('%s -- %s%s- %s Nexteer',NxtrConf,char(169),first,last)
      | end
  Data Store Write : DataStoreWrite  DataStoreName=NtcQlfr0X1D3
  Ground : Ground
  ISO Fault Debounce Design : Stateflow chart  TreatAsAtomicUnit=on
      settings: AttributesFormatString=|
      | Simulation Purpose Only.
      | Do Not Code this block
      | Diagnostic Manager Owns this requirement
  Terminator : Terminator
  Terminator1 : Terminator
  wires:
  NtcStInfo/1 -> Terminator1/1
  NtcNr/1 -> Terminator/1
  NtcSts/1 -> ISO Fault Debounce Design/1(NtcSts)
  DebStep/1 -> ISO Fault Debounce Design/2(DebStep)
  ISO Fault Debounce Design/1(Qualifier) -> Data Store Write/1
  Ground/1 -> ISO Fault Debounce Design/3(SvcClr)

== system ES105A_StHlthSigNormn/StHlthSigNormn/UpdRawSig/Current Error/NTC Sts Calculation/CopyRight2 ==

== system ES105A_StHlthSigNormn/StHlthSigNormn/UpdRawSig/Current Error/NTC Sts Calculation/NtcFaild ==
  Action Port : ActionPort  ActionType=then
  Constant2 : Constant  Value=NtcSts1.NTCSTS_FAILD  OutDataTypeStr=Enum: NtcSts1
  CopyRight2 : Subsystem  Description=|  mask(Copyright Information){none=on}
      | Copyright info block.                                               
      |                                                                     
      | Place copyright information at the top of every subsystem in design.
      mask prompts: none "No parameters"
      mask help: Place copyright information at the top of every subsystem in design.
      mask Display:
      | NxtrConf = 'Nexteer Confidential';
      | 
      | sys = bdroot; %handle for the current model ("system")
      | first = get_param(sys,'Created');
      | first = first(end-3:end);  %year is last four digits
      | 
      | last = get_param(sys,'LastModifiedDate');
      | if isempty(last)
      |     last = datestr(now,'yyyy');
      | else
      |     last = last(end-3:end);
      | end
      | 
      | if strcmp(first,last)
      |     fprintf('%s -- Copyright %s Nexteer',NxtrConf,first)
      | else
      |     fprintf('%s -- %s%s- %s Nexteer',NxtrConf,char(169),first,last)
      | end
  NtcFaild : Outport
  wires:
  Constant2/1 -> NtcFaild/1

== system ES105A_StHlthSigNormn/StHlthSigNormn/UpdRawSig/Current Error/NTC Sts Calculation/NtcPassd ==
  Action Port : ActionPort  ActionType=else
  Constant2 : Constant  Value=NtcSts1.NTCSTS_PASSD  OutDataTypeStr=Enum: NtcSts1
  CopyRight2 : Subsystem  Description=|  mask(Copyright Information){none=on}
      | Copyright info block.                                               
      |                                                                     
      | Place copyright information at the top of every subsystem in design.
      mask prompts: none "No parameters"
      mask help: Place copyright information at the top of every subsystem in design.
      mask Display:
      | NxtrConf = 'Nexteer Confidential';
      | 
      | sys = bdroot; %handle for the current model ("system")
      | first = get_param(sys,'Created');
      | first = first(end-3:end);  %year is last four digits
      | 
      | last = get_param(sys,'LastModifiedDate');
      | if isempty(last)
      |     last = datestr(now,'yyyy');
      | else
      |     last = last(end-3:end);
      | end
      | 
      | if strcmp(first,last)
      |     fprintf('%s -- Copyright %s Nexteer',NxtrConf,first)
      | else
      |     fprintf('%s -- %s%s- %s Nexteer',NxtrConf,char(169),first,last)
      | end
  NtcPassd : Outport
  wires:
  Constant2/1 -> NtcPassd/1

== system ES105A_StHlthSigNormn/StHlthSigNormn/UpdRawSig/Digital Torque Sensor /DigTqIdptSigStHlth Calc/CopyRight2 ==

== system ES105A_StHlthSigNormn/StHlthSigNormn/UpdRawSig/Digital Torque Sensor /DigTqIdptSigStHlth Calc/If Action Subsystem4 ==
  Action Port : ActionPort  ActionType=then
  Constant : Constant  Value=HLTH100PERC_CNT_U08
  CopyRight2 : Subsystem  Description=|  mask(Copyright Information){none=on}
      | Copyright info block.                                               
      |                                                                     
      | Place copyright information at the top of every subsystem in design.
      mask prompts: none "No parameters"
      mask help: Place copyright information at the top of every subsystem in design.
      mask Display:
      | NxtrConf = 'Nexteer Confidential';
      | 
      | sys = bdroot; %handle for the current model ("system")
      | first = get_param(sys,'Created');
      | first = first(end-3:end);  %year is last four digits
      | 
      | last = get_param(sys,'LastModifiedDate');
      | if isempty(last)
      |     last = datestr(now,'yyyy');
      | else
      |     last = last(end-3:end);
      | end
      | 
      | if strcmp(first,last)
      |     fprintf('%s -- Copyright %s Nexteer',NxtrConf,first)
      | else
      |     fprintf('%s -- %s%s- %s Nexteer',NxtrConf,char(169),first,last)
      | end
  DigTqIdptSigStHlth : Outport
  wires:
  Constant/1 -> DigTqIdptSigStHlth/1

== system ES105A_StHlthSigNormn/StHlthSigNormn/UpdRawSig/Digital Torque Sensor /DigTqIdptSigStHlth Calc/If Action Subsystem5 ==
  HwTqIdptSig : Inport
  Action Port : ActionPort  ActionType=else
  Constant1 : Constant  Value=StHlthSigNormnIdptSigStHlthSca
  CopyRight2 : Subsystem  Description=|  mask(Copyright Information){none=on}
      | Copyright info block.                                               
      |                                                                     
      | Place copyright information at the top of every subsystem in design.
      mask prompts: none "No parameters"
      mask help: Place copyright information at the top of every subsystem in design.
      mask Display:
      | NxtrConf = 'Nexteer Confidential';
      | 
      | sys = bdroot; %handle for the current model ("system")
      | first = get_param(sys,'Created');
      | first = first(end-3:end);  %year is last four digits
      | 
      | last = get_param(sys,'LastModifiedDate');
      | if isempty(last)
      |     last = datestr(now,'yyyy');
      | else
      |     last = last(end-3:end);
      | end
      | 
      | if strcmp(first,last)
      |     fprintf('%s -- Copyright %s Nexteer',NxtrConf,first)
      | else
      |     fprintf('%s -- %s%s- %s Nexteer',NxtrConf,char(169),first,last)
      | end
  Data Type Conversion : DataTypeConversion  OutDataTypeStr=uint8
  Product : Product
  DigTqIdptSigStHlth : Outport
  wires:
  HwTqIdptSig/1 -> Product/1
  Constant1/1 -> Product/2
  Product/1 -> Data Type Conversion/1
  Data Type Conversion/1 -> DigTqIdptSigStHlth/1

== system ES105A_StHlthSigNormn/StHlthSigNormn/UpdRawSig/Digital Torque Sensor /DigTqSnsrAStHlth Calc/CopyRight2 ==

== system ES105A_StHlthSigNormn/StHlthSigNormn/UpdRawSig/Digital Torque Sensor /DigTqSnsrAStHlth Calc/If Action Subsystem ==
  Action Port : ActionPort  ActionType=then
  Constant : Constant  Value=HLTH0PERC_CNT_U08  OutDataTypeStr=uint8
  CopyRight2 : Subsystem  Description=|  mask(Copyright Information){none=on}
      | Copyright info block.                                               
      |                                                                     
      | Place copyright information at the top of every subsystem in design.
      mask prompts: none "No parameters"
      mask help: Place copyright information at the top of every subsystem in design.
      mask Display:
      | NxtrConf = 'Nexteer Confidential';
      | 
      | sys = bdroot; %handle for the current model ("system")
      | first = get_param(sys,'Created');
      | first = first(end-3:end);  %year is last four digits
      | 
      | last = get_param(sys,'LastModifiedDate');
      | if isempty(last)
      |     last = datestr(now,'yyyy');
      | else
      |     last = last(end-3:end);
      | end
      | 
      | if strcmp(first,last)
      |     fprintf('%s -- Copyright %s Nexteer',NxtrConf,first)
      | else
      |     fprintf('%s -- %s%s- %s Nexteer',NxtrConf,char(169),first,last)
      | end
  DigTqSnsrAStHlth : Outport
  wires:
  Constant/1 -> DigTqSnsrAStHlth/1
